simulink model "car_mode"  (Simulink 9.2)
settings: Solver=VariableStepAuto  StartTime=0.0  StopTime=600  RelTol=1e-3
settings Model: Creator=Administrator  LastModifiedBy=Administrator
settings DataIOCC: LimitDataPoints=off  SaveFormat=Dataset  SignalLoggingSaveFormat=Dataset
settings OptimizationCC: LifeSpan=auto
settings DebuggingCC: UnderspecifiedInitializationDetection=Simplified  MergeDetectMultiDrivingBlocksExec=error  FcnCallInpInsideContextMsg=error  StateNameClashWarn=none  SFUnexpectedBacktrackingDiag=error  SFNoUnconditionalDefaultTransitionDiag=error  SFExecutionAtInitializationDiag=warning
settings HardwareCC: ProdBitPerPointer=64  ProdBitPerSizeT=64  ProdBitPerPtrDiffT=64  ProdLargestAtomicFloat=Float  ProdIntDivRoundTo=Zero  ProdEndianess=LittleEndian  ProdWordSize=64  ProdHWDeviceType=Intel->x86-64 (Windows64)
settings ModelReferenceCC: PropagateSignalLabelsOutOfModel=on
settings SFSimCC: SimUseLocalCustomCode=on
settings RTWCC: RTWUseLocalCustomCode=on
settings CodeAppCC: StateflowObjectComments=off
settings GRTTargetCC: TargetLangStandard=C99 (ISO)  GeneratePreprocessorConditionals=Use local settings  CombineOutputUpdateFcns=on  GRTInterface=off
settings ConfigComp: CovMetricSettings=dwe  CovHtmlReporting=off  CovSaveCumulativeToWorkspaceVar=off  CovSaveSingleToWorkspaceVar=off  CovExternalEMLEnable=on

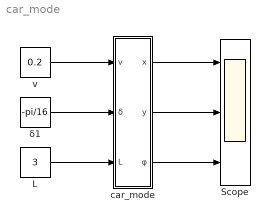
== system car_mode ==
  " L" : Constant  Value=3
  " δ1" : Constant  Value=-pi/16
  Scope : Scope  NumInputPorts=3
  "car_mode " : Subsystem
  v : Constant  Value=0.2
  wires:
  v/1 -> "car_mode "/1(v)
  "car_mode "/1("x ") -> Scope/1
  "car_mode "/2(y) -> Scope/2
  "car_mode "/3(φ) -> Scope/3
  " L"/1 -> "car_mode "/3(L)
  " δ1"/1 -> "car_mode "/2(δ)

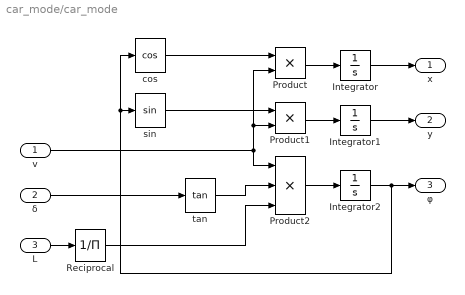
== system car_mode/car_mode  ==
  v : Inport
  δ : Inport  Port=2
  L : Inport  Port=3
  Integrator : Integrator
  Integrator1 : Integrator
  Integrator2 : Integrator  InitialCondition=pi/2
  Product : Product
  Product1 : Product
  Product2 : Product  Inputs=3
  Reciprocal : Product  Inputs=/
  cos : Trigonometry  Operator=cos
  sin : Trigonometry
  tan : Trigonometry  Operator=tan
  "x " : Outport
  y : Outport  Port=2
  φ : Outport  Port=3
  wires:
  cos/1 -> Product/1
  Integrator2/1 -> sin/1, cos/1, φ/1
  sin/1 -> Product1/1
  tan/1 -> Product2/2
  Product/1 -> Integrator/1
  Integrator1/1 -> y/1
  v/1 -> Product1/2, Product/2, Product2/1
  Product2/1 -> Integrator2/1
  Product1/1 -> Integrator1/1
  δ/1 -> tan/1
  Integrator/1 -> "x "/1
  L/1 -> Reciprocal/1
  Reciprocal/1 -> Product2/3
